simulink model "SignatureDemo"  (Simulink 7.8)
settings: Solver=ode3  StartTime=0.0  StopTime=10.0  RelTol=1e-3
settings Model: Creator=Jeff  LastModifiedBy=monika

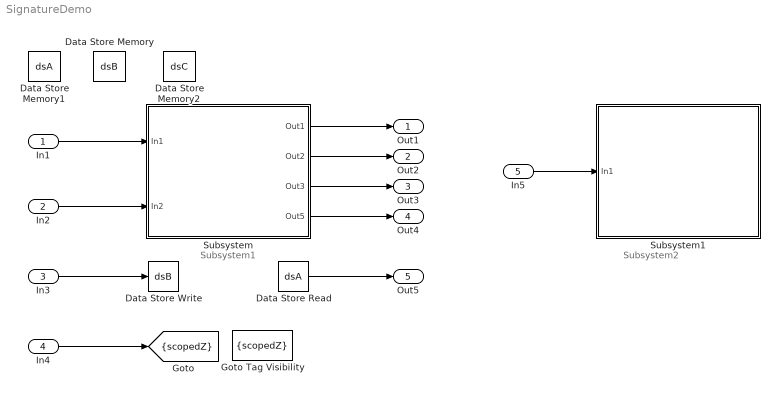
== system SignatureDemo ==
  note: Subsystem1
  note: Subsystem2
  In1 : Inport
  In2 : Inport  Port=2
  In3 : Inport  Port=3
  In4 : Inport  Port=4
  In5 : Inport  Port=5
  Data Store Memory : DataStoreMemory  DataStoreName=dsB  ReadBeforeWriteMsg=warning  WriteAfterWriteMsg=warning  WriteAfterReadMsg=warning
  Data Store Memory1 : DataStoreMemory  DataStoreName=dsA  ReadBeforeWriteMsg=warning  WriteAfterWriteMsg=warning  WriteAfterReadMsg=warning
  Data Store Memory2 : DataStoreMemory  DataStoreName=dsC  ReadBeforeWriteMsg=warning  WriteAfterWriteMsg=warning  WriteAfterReadMsg=warning
  Data Store Read : DataStoreRead  DataStoreName=dsA
  Data Store Write : DataStoreWrite  DataStoreName=dsB
  Goto Tag Visibility : GotoTagVisibility  GotoTag=scopedZ
  Subsystem : Subsystem
  Subsystem1 : Subsystem
  Out1 : Outport
  Out2 : Outport  Port=2
  Out3 : Outport  Port=3
  Out4 : Outport  Port=4
  Out5 : Outport  Port=5
  tag scope: scopedZ=scoped
  wires:
  In1/1 -> Subsystem/1(In1)
  In2/1 -> Subsystem/2(In2)
  In3/1 -> Data Store Write/1
  Subsystem/1(Out1) -> Out1/1
  Subsystem/2(Out2) -> Out2/1
  Subsystem/3(Out3) -> Out3/1
  Subsystem/4(Out5) -> Out4/1
  In4/1 -> [scopedZ]
  Data Store Read/1 -> Out5/1
  In5/1 -> Subsystem1/1(In1)

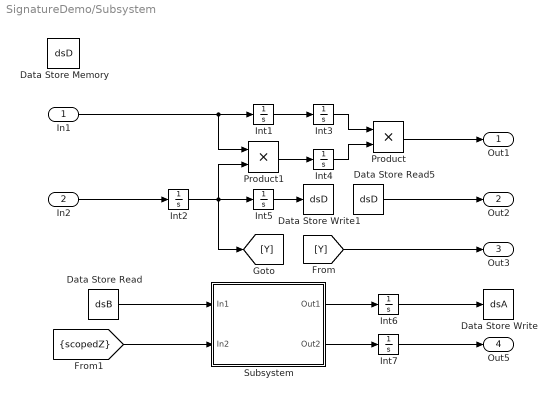
== system SignatureDemo/Subsystem ==
  In1 : Inport
  In2 : Inport  Port=2
  Data Store Memory : DataStoreMemory  DataStoreName=dsD  ReadBeforeWriteMsg=warning  WriteAfterWriteMsg=warning  WriteAfterReadMsg=warning
  Data Store Read : DataStoreRead  DataStoreName=dsB
  Data Store Read5 : DataStoreRead  DataStoreName=dsD
  Data Store Write : DataStoreWrite  DataStoreName=dsA
  Data Store Write1 : DataStoreWrite  DataStoreName=dsD
  Int{1..7} (7 alike) : Integrator
  Product : Product  RndMeth=Zero
  Product1 : Product  RndMeth=Zero
  Subsystem : Subsystem
  Out1 : Outport
  Out2 : Outport  Port=2
  Out3 : Outport  Port=3
  Out5 : Outport  Port=4
  wires:
  Int1/1 -> Int3/1
  Int3/1 -> Product/1
  Int4/1 -> Product/2
  Product1/1 -> Int4/1
  Int2/1 -> Product1/2, [Y], Int5/1
  Subsystem/1(Out1) -> Int6/1
  Subsystem/2(Out2) -> Int7/1
  [scopedZ] -> Subsystem/2(In2)
  Data Store Read/1 -> Subsystem/1(In1)
  Int6/1 -> Data Store Write/1
  Int5/1 -> Data Store Write1/1
  In1/1 -> Int1/1, Product1/1
  In2/1 -> Int2/1
  Product/1 -> Out1/1
  Data Store Read5/1 -> Out2/1
  [Y] -> Out3/1
  Int7/1 -> Out5/1

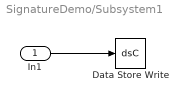
== system SignatureDemo/Subsystem1 ==
  In1 : Inport
  Data Store Write : DataStoreWrite  DataStoreName=dsC
  wires:
  In1/1 -> Data Store Write/1

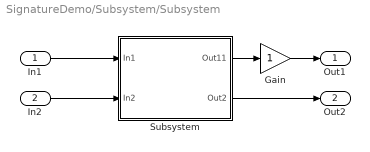
== system SignatureDemo/Subsystem/Subsystem ==
  In1 : Inport
  In2 : Inport  Port=2
  Gain : Gain
  Subsystem : Subsystem
  Out1 : Outport
  Out2 : Outport  Port=2
  wires:
  In1/1 -> Subsystem/1(In1)
  Subsystem/1(Out11) -> Gain/1
  In2/1 -> Subsystem/2(In2)
  Subsystem/2(Out2) -> Out2/1
  Gain/1 -> Out1/1

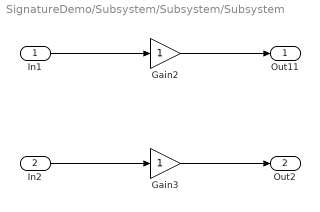
== system SignatureDemo/Subsystem/Subsystem/Subsystem ==
  In1 : Inport
  In2 : Inport  Port=2
  Gain2 : Gain
  Gain3 : Gain
  Out11 : Outport
  Out2 : Outport  Port=2
  wires:
  In1/1 -> Gain2/1
  In2/1 -> Gain3/1
  Gain2/1 -> Out11/1
  Gain3/1 -> Out2/1
